simulink model "ex_25_model_f2"  (R2014a)
settings: Solver=ode45  StartTime=0.0  StopTime=0.5  RelTol=1e-3
values from neighbouring files (symbols this model uses):
  Kp = Kp*10    [ex_25_plots.m]
undefined symbols (not defined in the file or in its folder): ki, x, y, z
settings Model: Creator=Nino  LastModifiedBy=Nino

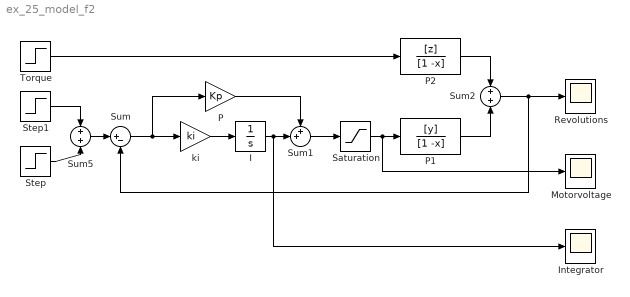
== system ex_25_model_f2 ==
  I : Integrator
  Integrator : Scope
      settings: YMin=0.9989  YMax=0.9999  SaveName=Integrator
  "Motorvoltage " : Scope
      settings: YMin=0.9989  YMax=0.9999  SaveName=Motorvoltage
  P : Gain  Gain=Kp
  P1 : TransferFcn  Numerator=[y]  Denominator=[1 -x]
  P2 : TransferFcn  Numerator=[z]  Denominator=[1 -x]
  Revolutions : Scope
      settings: YMin=0.9989  YMax=0.9999  SaveName=Revolutions
  Saturation : Saturate  UpperLimit=10  LowerLimit=-10  LinearizeAsGain=off
  Step : Step  Time=0.1  After=-1000  SampleTime=0
  Step1 : Step  Time=0  After=1000  SampleTime=0
  Sum : Sum  Inputs=|+-
  Sum1 : Sum  Inputs=++|
  Sum2 : Sum  Inputs=+|+
  Sum5 : Sum  Inputs=+|+
  Torque : Step  Time=100  After=0  SampleTime=0
  ki : Gain  Gain=ki
  wires:
  P2/1 -> Sum2/1
  Sum2/1 -> Sum/2, Revolutions/1
  ki/1 -> I/1
  Sum/1 -> P/1, ki/1
  P/1 -> Sum1/1
  I/1 -> Integrator/1, Sum1/2
  P1/1 -> Sum2/2
  Saturation/1 -> "Motorvoltage "/1, P1/1
  Sum1/1 -> Saturation/1
  Torque/1 -> P2/1
  Step1/1 -> Sum5/1
  Step/1 -> Sum5/2
  Sum5/1 -> Sum/1
